simulink model "Current_Regulator"  (R2015a)
settings: Solver=ode5  StartTime=0.0  StopTime=10  FixedStep=Ts  RelTol=1e-3
InitFcn:
  | %==========================================================================
  | %% INIT FUNCTION FOR CURRENT REGULATOR
  | close all; clear all; clc;
  | 
  | iq_int_error = 0;
  | id_int_error = 0;
  | theta = 0;
  | P = 8;
  | Jp = 1.9e-5;
  | 
  | Ts = 1/20000;
  | Ts_motion = 1/2000;
  | 
  | Kp = 0.6283;%0.9463;%
  | Ki = 1131;%3.3149e5;%
  | 
  | K1 = 679.3446;
  | K2 = 38804.0;
  | K3 = 0.772497214924591;
  | K4 = 2354.393299072175;
  | 
  | ba   = 0.0071213;
  | Ksa  = 0.455;
  | Kisa = 4.5045;
  | 
  | Rs = 0.72/sqrt(3);
  | Ld = 0.4e-3/sqrt(3);
  | Lq = Ld;
  | tau = Lq/Rs;
  | gam = exp(-Ts/tau);
  | del = 1-gam;
  | lambda_pm = 0.0067;
  | 
  | we = 500;
libraries: dspsrcs4 x3, simulink x1
settings Model: Creator=RDL  LastModifiedBy=RDL

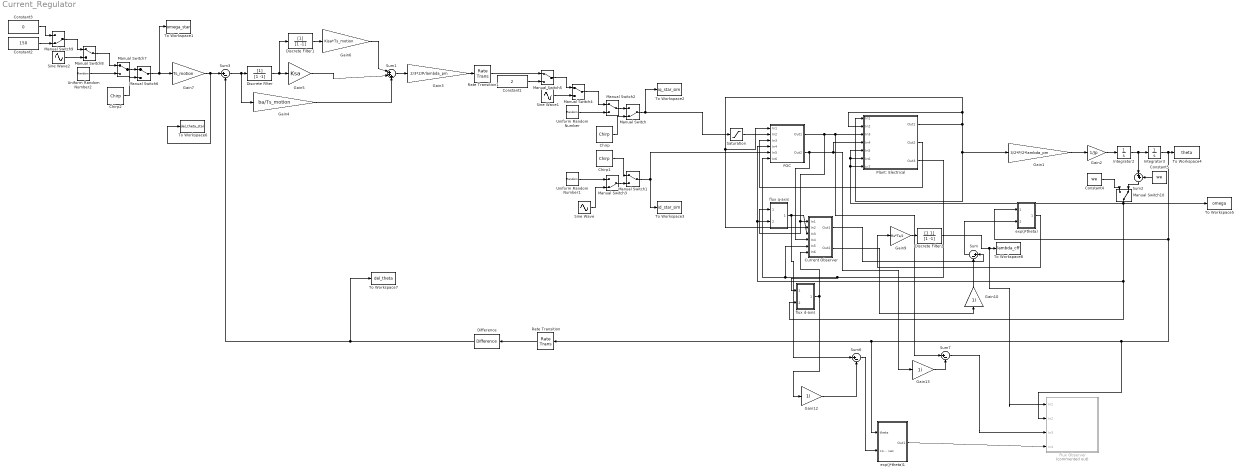
== system Current_Regulator ==
  Chirp : dspsrcs4/Chirp  sweep=Linear  mode=Unidirectional  f0=0.1  f1=10000  t1=1  Tsweep=1  phase=pi/2  Ts=Ts  spf=1  datatype=Double
  Chirp1 : dspsrcs4/Chirp  sweep=Linear  mode=Unidirectional  f0=0.1  f1=10000  t1=1  Tsweep=1  phase=0  Ts=Ts  spf=1  datatype=Double
  Chirp2 : dspsrcs4/Chirp  sweep=Linear  mode=Unidirectional  f0=0.1  f1=1000  t1=1  Tsweep=1  phase=0  Ts=Ts_motion  spf=1  datatype=Double
  Constant1 : Constant  Value=2
  Constant2 : Constant  Value=150  SampleTime=Ts_motion
  Constant3 : Constant  Value=0  SampleTime=Ts_motion
  Constant4 : Constant  Value=we
  Constant5 : Constant  Value=we
  Current Observer : Subsystem
  Difference : simulink/Discrete/Difference  ICPrevInput=0.0  InputProcessing=Inherited  OutMin=[]  OutMax=[]  OutDataType=fixdt(1, 16)  OutScaling=2^-10  DoSatur=off
  Discrete Filter : DiscreteFilter  Denominator=[1 -1]
  Discrete Filter1 : DiscreteFilter  Denominator=[1 -1]
  Discrete Filter2 : DiscreteFilter  Numerator=[1 1]  Denominator=[1 -1]  SampleTime=Ts
  FOC : Subsystem
  Flux Observer : Subsystem  Commented=on
  Gain1 : Gain  Gain=3/2*P/2*lambda_pm
  Gain10 : Gain  Gain=1i
  Gain12 : Gain  Gain=1i
  Gain13 : Gain  Gain=1i
  Gain2 : Gain  Gain=1/Jp
  Gain3 : Gain  Gain=2/3*2/P/lambda_pm
  Gain4 : Gain  Gain=ba/Ts_motion
  Gain5 : Gain  Gain=Ksa
  Gain6 : Gain  Gain=Kisa*Ts_motion
  Gain7 : Gain  Gain=Ts_motion
  Gain9 : Gain  Gain=Rs*Ts/2
  Integrator2 : Integrator
  Integrator3 : Integrator
  Manual Switch{,3,9..10} (4 alike) : ManualSwitch  CurrentSetting=0
  Manual Switch{1..2,4..8} (7 alike) : ManualSwitch
  Plant: Electrical : Subsystem
  Rate Transition : RateTransition  OutPortSampleTime=Ts_motion
  Rate Transition1 : RateTransition  OutPortSampleTime=Ts
  Saturation : Saturate  UpperLimit=5  LowerLimit=-5
  Sine Wave : Sin  Amplitude=0  Frequency=2*pi*8  SampleTime=Ts
  Sine Wave1 : Sin  Amplitude=0.8  Frequency=2*pi*24  Phase=pi/2  SampleTime=Ts
  Sine Wave2 : Sin  Amplitude=0.8  Frequency=2*pi*24  Phase=pi/2  SampleTime=Ts_motion
  Sum{,3,6..7} (4 alike) : Sum  Inputs=|+-
  Sum1 : Sum  Inputs=|+++
  Sum2 : Sum  Inputs=|++
  To Workspace1 : ToWorkspace  VariableName=omega_star  SaveFormat=Timeseries  SampleTime=-1
  To Workspace2 : ToWorkspace  VariableName=iq_star_sim  SaveFormat=Timeseries  SampleTime=-1
  To Workspace3 : ToWorkspace  VariableName=id_star_sim  SaveFormat=Timeseries  SampleTime=-1
  To Workspace4 : ToWorkspace  VariableName=theta  SaveFormat=Timeseries  SampleTime=-1
  To Workspace5 : ToWorkspace  VariableName=omega  SaveFormat=Timeseries  SampleTime=-1
  To Workspace6 : ToWorkspace  VariableName=del_theta_star  SaveFormat=Timeseries  SampleTime=-1
  To Workspace7 : ToWorkspace  VariableName=del_theta  SaveFormat=Timeseries  SampleTime=-1
  To Workspace8 : ToWorkspace  VariableName=lambda_cff  SaveFormat=Timeseries  SampleTime=-1
  Uniform Random Number : UniformRandomNumber  Minimum=-5  Maximum=5  Seed=1  SampleTime=Ts
  Uniform Random Number1 : UniformRandomNumber  Minimum=-5  Maximum=5  SampleTime=Ts
  Uniform Random Number2 : UniformRandomNumber  Minimum=-5  Maximum=5  Seed=1  SampleTime=Ts_motion
  exp(j*theta) : Subsystem
  exp(j*theta)1 : Subsystem
  flux d-axis : Subsystem
  flux q-axis : Subsystem
  wires:
  Integrator2/1 -> Sum2/1, Integrator3/1
  Manual Switch/1 -> Saturation/1, To Workspace2/1
  Manual Switch1/1 -> FOC/5(In5), To Workspace3/1
  Manual Switch2/1 -> Manual Switch/1
  Manual Switch3/1 -> Manual Switch1/2
  Chirp1/1 -> Manual Switch1/1
  Chirp/1 -> Manual Switch/2
  Uniform Random Number/1 -> Manual Switch2/2
  Uniform Random Number1/1 -> Manual Switch3/1
  Sine Wave/1 -> Manual Switch3/2
  Gain1/1 -> Gain2/1
  Gain2/1 -> Integrator2/1
  Integrator3/1 -> exp(j*theta)/1(In1), Flux Observer/2(In2), exp(j*theta)1/1(theta), Rate Transition/1, To Workspace4/1
  Manual Switch4/1 -> Manual Switch2/1
  Sine Wave1/1 -> Manual Switch4/2
  Plant: Electrical/1(Out1) -> Current Observer/2(In2), FOC/1(In1), Plant: Electrical/2(In2), Gain1/1, Plant: Electrical/1(In1)
  FOC/1(Out1) -> flux q-axis/1(In1), Current Observer/1(In1), Sum7/1, Plant: Electrical/3(In3)
  FOC/2(Out2) -> Current Observer/4(In4), Gain13/1, Plant: Electrical/4(In4)
  Plant: Electrical/2(Out2) -> FOC/3(In3)
  Plant: Electrical/3(Out3) -> flux d-axis/1(In1), Current Observer/5(In5), FOC/6(In6)
  Manual Switch5/1 -> Manual Switch4/1
  Constant1/1 -> Manual Switch5/2
  Gain3/1 -> Rate Transition1/1
  Rate Transition/1 -> Difference/1
  Difference/1 -> To Workspace7/1, Sum3/2
  Gain4/1 -> Sum1/3
  Sum3/1 -> Discrete Filter/1, Gain4/1
  Discrete Filter/1 -> Discrete Filter1/1, Gain5/1
  Gain5/1 -> Sum1/2
  Discrete Filter1/1 -> Gain6/1
  Gain6/1 -> Sum1/1
  Sum1/1 -> Gain3/1
  Manual Switch7/1 -> Manual Switch6/1
  Chirp2/1 -> Manual Switch6/2
  Uniform Random Number2/1 -> Manual Switch7/2
  Manual Switch8/1 -> Manual Switch7/1
  Sine Wave2/1 -> Manual Switch8/2
  Manual Switch9/1 -> Manual Switch8/1
  Constant2/1 -> Manual Switch9/2
  Manual Switch6/1 -> To Workspace1/1, Gain7/1
  Gain7/1 -> To Workspace6/1, Sum3/1
  Rate Transition1/1 -> Manual Switch5/1
  Saturation/1 -> FOC/2(In2)
  flux d-axis/1(Out1) -> Current Observer/6(In6), Gain12/1
  flux q-axis/1(Out1) -> Sum6/1, Current Observer/3(In3)
  Current Observer/1(Out1) -> Sum/1
  Current Observer/2(Out2) -> Gain10/1
  Constant3/1 -> Manual Switch9/1
  Constant4/1 -> Manual Switch10/1
  Manual Switch10/1 -> FOC/4(In4), flux q-axis/2(In2), flux d-axis/2(In2), To Workspace5/1, Plant: Electrical/7(In7), Plant: Electrical/6(In6), Plant: Electrical/5(In5)
  Gain9/1 -> Discrete Filter2/1
  Gain10/1 -> Sum/2
  Discrete Filter2/1 -> Flux Observer/1(In1), To Workspace8/1
  Sum2/1 -> Manual Switch10/2
  Constant5/1 -> Sum2/2
  Sum/1 -> exp(j*theta)/2(In2)
  exp(j*theta)/1(Out1) -> Gain9/1
  Gain12/1 -> Sum6/2
  Gain13/1 -> Sum7/2
  Sum7/1 -> Flux Observer/3(In3)
  exp(j*theta)1/1(Out1) -> Flux Observer/4(In4)
  Sum6/1 -> exp(j*theta)1/2(complex vec)

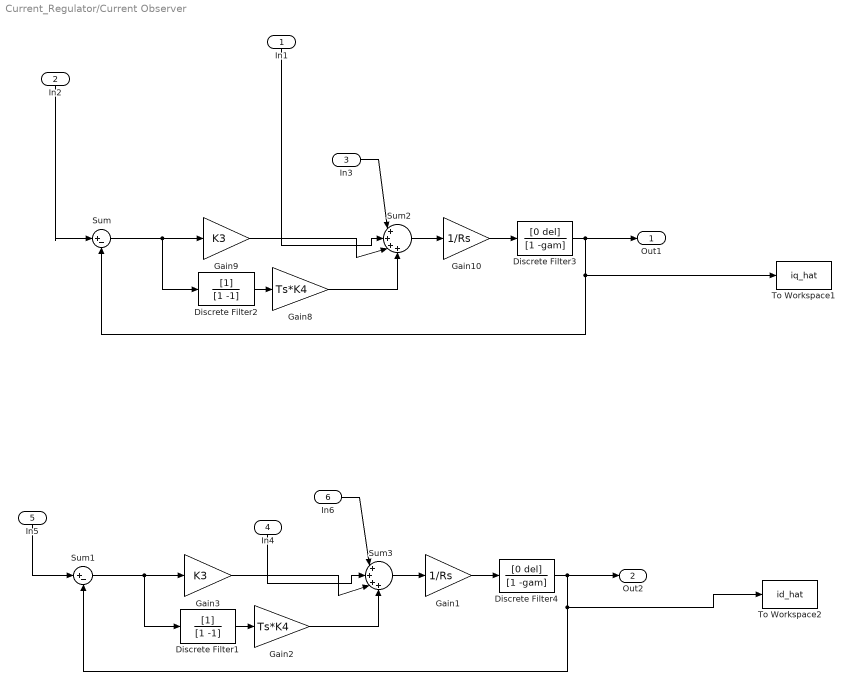
== system Current_Regulator/Current Observer ==
  In1 : Inport
  In2 : Inport  Port=2
  In3 : Inport  Port=3
  In4 : Inport  Port=4
  In5 : Inport  Port=5
  In6 : Inport  Port=6
  Discrete Filter1 : DiscreteFilter  Denominator=[1 -1]  SampleTime=Ts
  Discrete Filter2 : DiscreteFilter  Denominator=[1 -1]  SampleTime=Ts
  Discrete Filter3 : DiscreteFilter  Numerator=[0 del]  Denominator=[1 -gam]  SampleTime=Ts
  Discrete Filter4 : DiscreteFilter  Numerator=[0 del]  Denominator=[1 -gam]  SampleTime=Ts
  Gain1 : Gain  Gain=1/Rs
  Gain10 : Gain  Gain=1/Rs
  Gain2 : Gain  Gain=Ts*K4
  Gain3 : Gain  Gain=K3
  Gain8 : Gain  Gain=Ts*K4
  Gain9 : Gain  Gain=K3
  Sum : Sum  Inputs=|+-
  Sum1 : Sum  Inputs=|+-
  Sum2 : Sum  Inputs=|++++
  Sum3 : Sum  Inputs=|++++
  To Workspace1 : ToWorkspace  VariableName=iq_hat  SaveFormat=Timeseries  SampleTime=-1
  To Workspace2 : ToWorkspace  VariableName=id_hat  SaveFormat=Timeseries  SampleTime=-1
  Out1 : Outport
  Out2 : Outport  Port=2
  wires:
  Discrete Filter2/1 -> Gain8/1
  Gain9/1 -> Sum2/3
  Sum/1 -> Discrete Filter2/1, Gain9/1
  Gain10/1 -> Discrete Filter3/1
  In3/1 -> Sum2/1
  Discrete Filter3/1 -> Out1/1, Sum/2, To Workspace1/1
  Sum2/1 -> Gain10/1
  Gain8/1 -> Sum2/4
  In2/1 -> Sum/1
  In1/1 -> Sum2/2
  Discrete Filter1/1 -> Gain2/1
  Gain3/1 -> Sum3/3
  Sum1/1 -> Discrete Filter1/1, Gain3/1
  Gain1/1 -> Discrete Filter4/1
  In6/1 -> Sum3/1
  Discrete Filter4/1 -> Out2/1, To Workspace2/1, Sum1/2
  Sum3/1 -> Gain1/1
  Gain2/1 -> Sum3/4
  In5/1 -> Sum1/1
  In4/1 -> Sum3/2

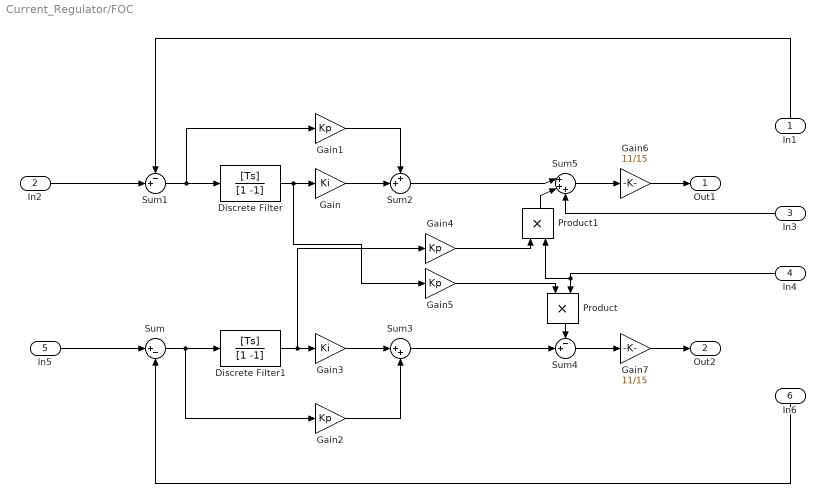
== system Current_Regulator/FOC ==
  In1 : Inport
  In2 : Inport  Port=2
  In3 : Inport  Port=3
  In4 : Inport  Port=4
  In5 : Inport  Port=5
  In6 : Inport  Port=6
  Discrete Filter : DiscreteFilter  Numerator=[Ts]  Denominator=[1 -1]  SampleTime=Ts
  Discrete Filter1 : DiscreteFilter  Numerator=[Ts]  Denominator=[1 -1]  SampleTime=Ts
  Gain : Gain  Gain=Ki
  Gain{1..2,4..5} (4 alike) : Gain  Gain=Kp
  Gain3 : Gain  Gain=Ki
  Gain6 : Gain  Gain=11/15
  Gain7 : Gain  Gain=11/15
  Product : Product
  Product1 : Product
  Sum : Sum  Inputs=|+-
  Sum1 : Sum  Inputs=-+|
  Sum2 : Sum  Inputs=++|
  Sum3 : Sum  Inputs=|++
  Sum4 : Sum  Inputs=-+|
  Sum5 : Sum  Inputs=|+++
  Out1 : Outport
  Out2 : Outport  Port=2
  wires:
  Sum1/1 -> Gain1/1, Discrete Filter/1
  Sum/1 -> Gain2/1, Discrete Filter1/1
  Discrete Filter/1 -> Gain5/1, Gain/1
  Gain/1 -> Sum2/2
  Gain1/1 -> Sum2/1
  Discrete Filter1/1 -> Gain4/1, Gain3/1
  Gain3/1 -> Sum3/1
  Gain2/1 -> Sum3/2
  Sum3/1 -> Sum4/2
  Sum2/1 -> Sum5/1
  Sum5/1 -> Gain6/1
  Product1/1 -> Sum5/2
  Gain4/1 -> Product1/1
  Product/1 -> Sum4/1
  Gain5/1 -> Product/1
  Sum4/1 -> Gain7/1
  In4/1 -> Product1/2, Product/2
  In1/1 -> Sum1/1
  In6/1 -> Sum/2
  In2/1 -> Sum1/2
  In3/1 -> Sum5/3
  In5/1 -> Sum/1
  Gain6/1 -> Out1/1
  Gain7/1 -> Out2/1

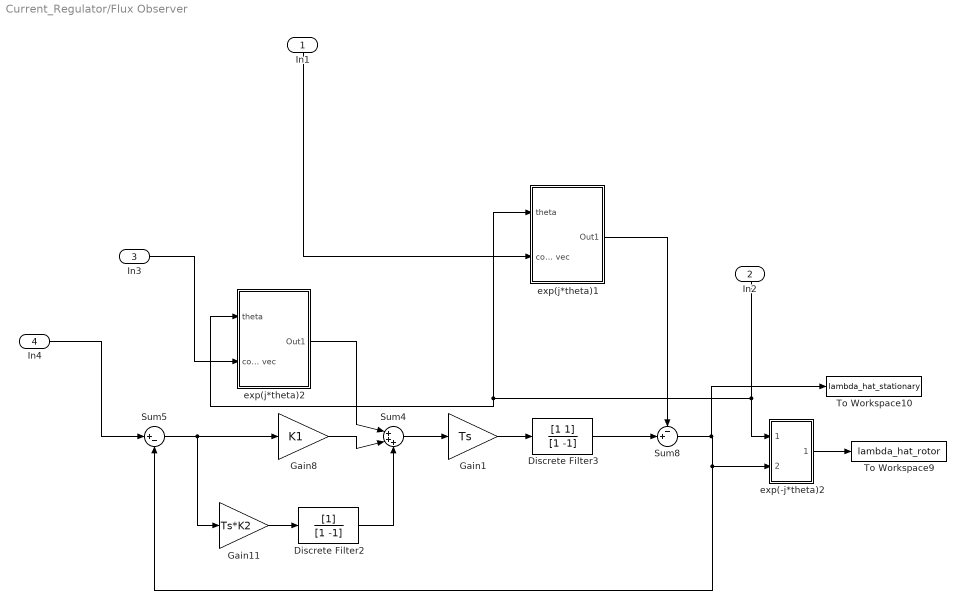
== system Current_Regulator/Flux Observer ==
  In1 : Inport
  In2 : Inport  Port=2
  In3 : Inport  Port=3
  In4 : Inport  Port=4
  Discrete Filter2 : DiscreteFilter  Denominator=[1 -1]  SampleTime=Ts
  Discrete Filter3 : DiscreteFilter  Numerator=[1 1]  Denominator=[1 -1]  SampleTime=Ts
  Gain1 : Gain  Gain=Ts
  Gain11 : Gain  Gain=Ts*K2  OutDataTypeStr=Inherit: Same as input
  Gain8 : Gain  Gain=K1
  Sum4 : Sum  Inputs=|+++
  Sum5 : Sum  Inputs=|+-
  Sum8 : Sum  Inputs=-+|
  To Workspace10 : ToWorkspace  VariableName=lambda_hat_stationary  SaveFormat=Timeseries  SampleTime=-1
  To Workspace9 : ToWorkspace  VariableName=lambda_hat_rotor  SaveFormat=Timeseries  SampleTime=-1
  exp(-j*theta)2 : Subsystem
  exp(j*theta)1 : Subsystem
  exp(j*theta)2 : Subsystem
  wires:
  Discrete Filter2/1 -> Sum4/3
  exp(-j*theta)2/1(Out1) -> To Workspace9/1
  Discrete Filter3/1 -> Sum8/2
  Sum8/1 -> To Workspace10/1, exp(-j*theta)2/2(In2), Sum5/2
  Gain11/1 -> Discrete Filter2/1
  Gain8/1 -> Sum4/2
  Sum5/1 -> Gain11/1, Gain8/1
  In4/1 -> Sum5/1
  In2/1 -> exp(j*theta)1/1(theta), exp(j*theta)2/1(theta), exp(-j*theta)2/1(In1)
  Gain1/1 -> Discrete Filter3/1
  Sum4/1 -> Gain1/1
  In1/1 -> exp(j*theta)1/2(complex vec)
  exp(j*theta)1/1(Out1) -> Sum8/1
  exp(j*theta)2/1(Out1) -> Sum4/1
  In3/1 -> exp(j*theta)2/2(complex vec)

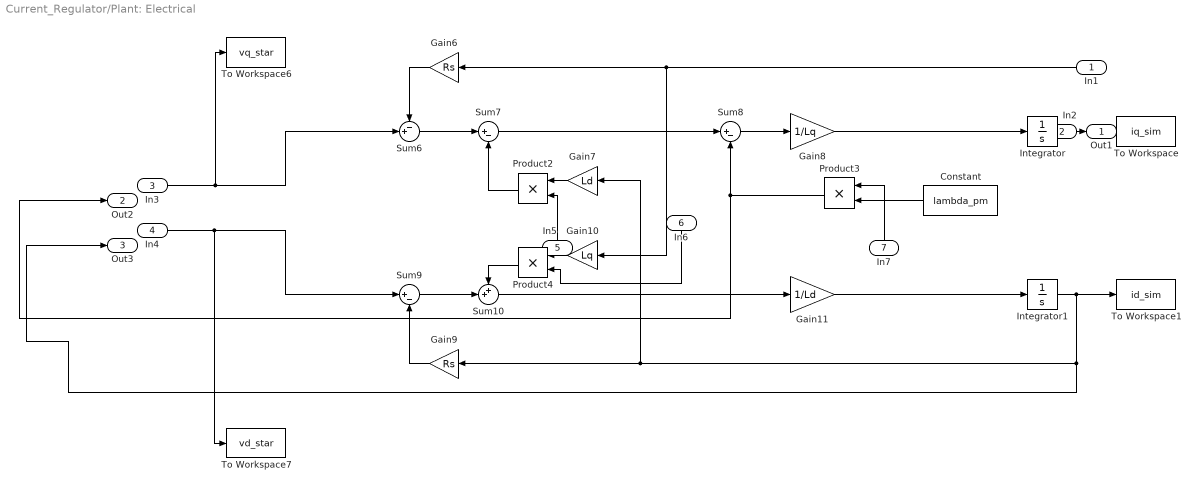
== system Current_Regulator/Plant: Electrical ==
  In1 : Inport
  In2 : Inport  Port=2
  In3 : Inport  Port=3
  In4 : Inport  Port=4
  In5 : Inport  Port=5
  In6 : Inport  Port=6
  In7 : Inport  Port=7
  Constant : Constant  Value=lambda_pm
  Gain10 : Gain  Gain=Lq
  Gain11 : Gain  Gain=1/Ld
  Gain6 : Gain  Gain=Rs
  Gain7 : Gain  Gain=Ld
  Gain8 : Gain  Gain=1/Lq
  Gain9 : Gain  Gain=Rs
  Integrator : Integrator
  Integrator1 : Integrator
  Product2 : Product
  Product3 : Product
  Product4 : Product
  Sum10 : Sum  Inputs=++|
  Sum6 : Sum  Inputs=-+|
  Sum7 : Sum  Inputs=|+-
  Sum8 : Sum  Inputs=|+-
  Sum9 : Sum  Inputs=|+-
  To Workspace : ToWorkspace  VariableName=iq_sim  SaveFormat=Timeseries  SampleTime=-1
  To Workspace1 : ToWorkspace  VariableName=id_sim  SaveFormat=Timeseries  SampleTime=-1
  To Workspace6 : ToWorkspace  VariableName=vq_star  SaveFormat=Timeseries  SampleTime=-1
  To Workspace7 : ToWorkspace  VariableName=vd_star  SaveFormat=Timeseries  SampleTime=-1
  Out1 : Outport
  Out2 : Outport  Port=2
  Out3 : Outport  Port=3
  wires:
  Gain6/1 -> Sum6/1
  Sum6/1 -> Sum7/1
  Gain7/1 -> Product2/1
  Product2/1 -> Sum7/2
  Constant/1 -> Product3/2
  Sum7/1 -> Sum8/1
  Sum8/1 -> Gain8/1
  Gain8/1 -> Integrator/1
  Integrator/1 -> Out1/1
  Sum9/1 -> Sum10/2
  Gain9/1 -> Sum9/2
  Gain10/1 -> Product4/1
  Product4/1 -> Sum10/1
  Sum10/1 -> Gain11/1
  Gain11/1 -> Integrator1/1
  Integrator1/1 -> To Workspace1/1, Out3/1, Gain7/1, Gain9/1
  Product3/1 -> Out2/1, Sum8/2
  In3/1 -> To Workspace6/1, Sum6/2
  In4/1 -> To Workspace7/1, Sum9/1
  In7/1 -> Product3/1
  In6/1 -> Product4/2
  In5/1 -> Product2/2
  In2/1 -> To Workspace/1
  In1/1 -> Gain6/1, Gain10/1

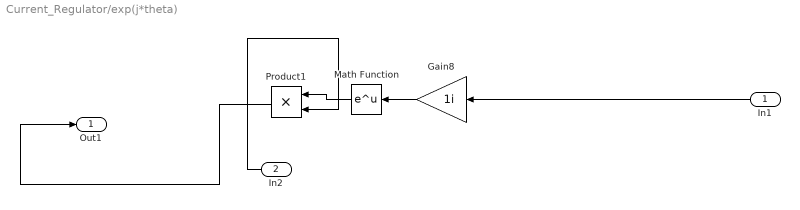
== system Current_Regulator/exp(j*theta) ==
  In1 : Inport
  In2 : Inport  Port=2
  Gain8 : Gain  Gain=1i
  Math Function : Math  OutputSignalType=complex  SaturateOnIntegerOverflow=on
  Product1 : Product
  Out1 : Outport
  wires:
  In1/1 -> Gain8/1
  Gain8/1 -> Math Function/1
  Math Function/1 -> Product1/1
  In2/1 -> Product1/2
  Product1/1 -> Out1/1

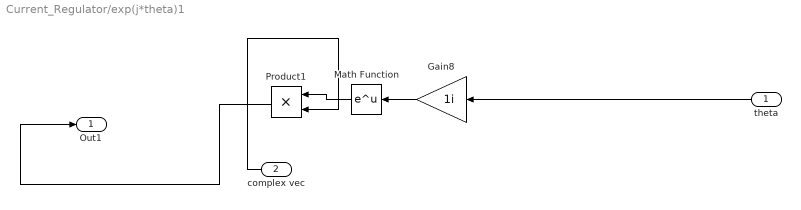
== system Current_Regulator/exp(j*theta)1 ==
  theta : Inport
  complex vec : Inport  Port=2
  Gain8 : Gain  Gain=1i
  Math Function : Math  OutputSignalType=complex  SaturateOnIntegerOverflow=on
  Product1 : Product
  Out1 : Outport
  wires:
  Product1/1 -> Out1/1
  complex vec/1 -> Product1/2
  Math Function/1 -> Product1/1
  Gain8/1 -> Math Function/1
  theta/1 -> Gain8/1

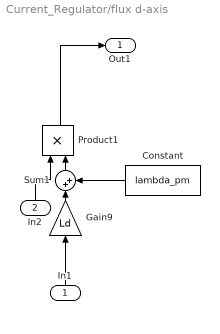
== system Current_Regulator/flux d-axis ==
  In1 : Inport
  In2 : Inport  Port=2
  Constant : Constant  Value=lambda_pm
  Gain9 : Gain  Gain=Ld
  Product1 : Product
  Sum1 : Sum  Inputs=|++
  Out1 : Outport
  wires:
  Product1/1 -> Out1/1
  Constant/1 -> Sum1/2
  In1/1 -> Gain9/1
  In2/1 -> Product1/1
  Sum1/1 -> Product1/2
  Gain9/1 -> Sum1/1

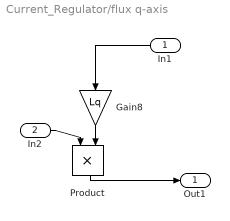
== system Current_Regulator/flux q-axis ==
  In1 : Inport
  In2 : Inport  Port=2
  Gain8 : Gain  Gain=Lq
  Product : Product
  Out1 : Outport
  wires:
  Product/1 -> Out1/1
  In2/1 -> Product/1
  In1/1 -> Gain8/1
  Gain8/1 -> Product/2

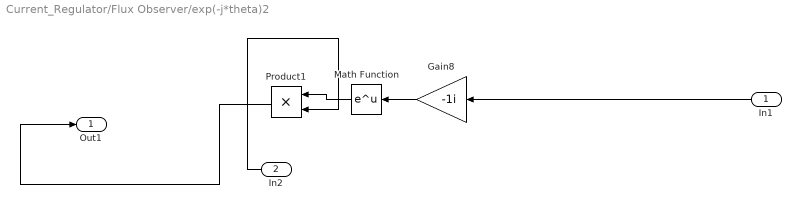
== system Current_Regulator/Flux Observer/exp(-j*theta)2 ==
  In1 : Inport
  In2 : Inport  Port=2
  Gain8 : Gain  Gain=-1i
  Math Function : Math  OutputSignalType=complex  SaturateOnIntegerOverflow=on
  Product1 : Product
  Out1 : Outport
  wires:
  In1/1 -> Gain8/1
  Gain8/1 -> Math Function/1
  Math Function/1 -> Product1/1
  In2/1 -> Product1/2
  Product1/1 -> Out1/1

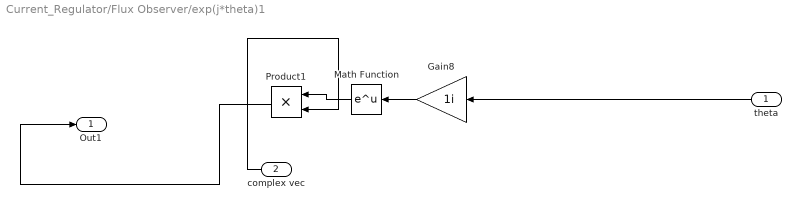
== system Current_Regulator/Flux Observer/exp(j*theta)1 ==
  theta : Inport
  complex vec : Inport  Port=2
  Gain8 : Gain  Gain=1i
  Math Function : Math  OutputSignalType=complex  SaturateOnIntegerOverflow=on
  Product1 : Product
  Out1 : Outport
  wires:
  Product1/1 -> Out1/1
  complex vec/1 -> Product1/2
  Math Function/1 -> Product1/1
  Gain8/1 -> Math Function/1
  theta/1 -> Gain8/1

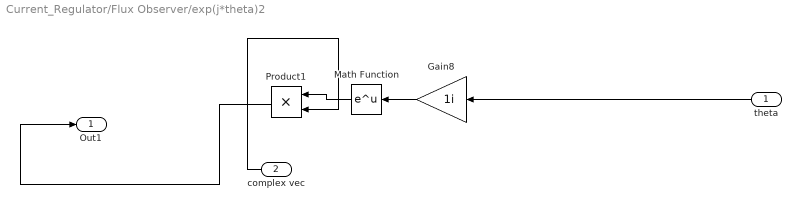
== system Current_Regulator/Flux Observer/exp(j*theta)2 ==
  theta : Inport
  complex vec : Inport  Port=2
  Gain8 : Gain  Gain=1i
  Math Function : Math  OutputSignalType=complex  SaturateOnIntegerOverflow=on
  Product1 : Product
  Out1 : Outport
  wires:
  theta/1 -> Gain8/1
  Gain8/1 -> Math Function/1
  Math Function/1 -> Product1/1
  complex vec/1 -> Product1/2
  Product1/1 -> Out1/1
